simulink model "Modelo2"  (R2020a)
settings: Solver=VariableStepAuto  StartTime=0.0  StopTime=inf  RelTol=1e-3
values from neighbouring files (symbols this model uses):
  A = [0        1    0       0 ... (first row only)    [PantografoSimulink.m]    (also in PantografoStep.m)
  B = [0 0 0 1/m2]'    [PantografoSimulink.m]    (also in PantografoStep.m)
  C = [1 0 0 0 ... (first row only)    [PantografoSimulink.m]    (also in PantografoStep.m)
  D = [0 0]'    [PantografoSimulink.m]    (also in PantografoStep.m)
settings Model: Creator=Androx  LastModifiedBy=Usuario

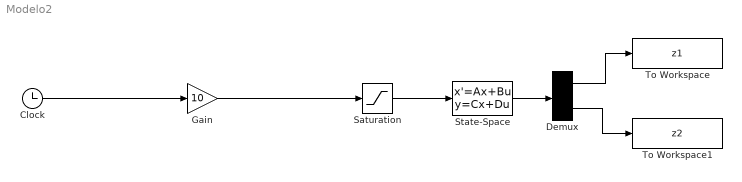
== system Modelo2 ==
  Clock : Clock
  Demux : Demux  Outputs=2
  Gain : Gain  Gain=10
  Saturation : Saturate  UpperLimit=2.2e6  LowerLimit=0
  State-Space : StateSpace  A=A  B=B  C=C  D=D  InitialCondition=zeros(4,1)
  To Workspace : ToWorkspace  VariableName=z1  SaveFormat=Timeseries  SampleTime=-1
  To Workspace1 : ToWorkspace  VariableName=z2  SaveFormat=Timeseries  SampleTime=-1
  wires:
  Saturation/1 -> State-Space/1
  State-Space/1 -> Demux/1
  Demux/1 -> To Workspace/1
  Demux/2 -> To Workspace1/1
  Gain/1 -> Saturation/1
  Clock/1 -> Gain/1
